simulink model "BPSK_EXP3"  (R2020a)
settings: Solver=VariableStepAuto  StartTime=0.0  StopTime=15  RelTol=1e-3
libraries: commrandsrc3 x1, dsparch4 x1
settings Model: Creator=User  LastModifiedBy=Raksha

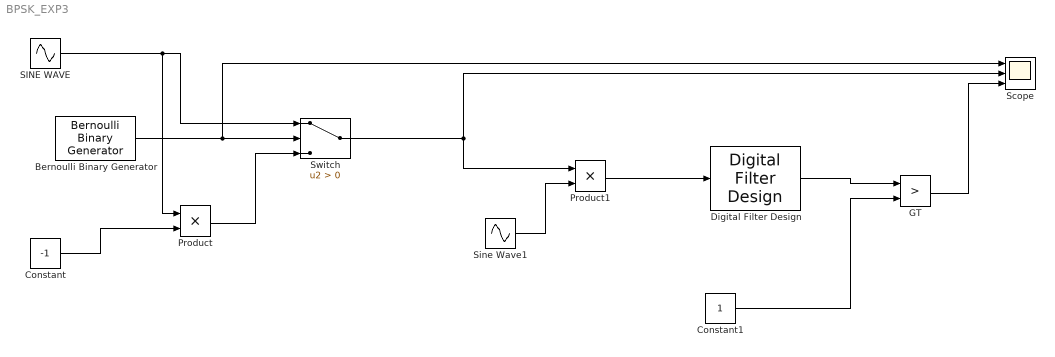
== system BPSK_EXP3 ==
  Bernoulli Binary Generator : commrandsrc3/Bernoulli Binary Generator  ProbabilityOfZero=0.5  SeedSource=Auto  Seed=0  SampleTime=1  SamplesPerFrame=1  OutputDataType=double  SimulateUsing=Interpreted execution
  Constant : Constant  Value=-1
  Constant1 : Constant
  Digital Filter Design : dsparch4/Digital Filter Design  mwdsp_browser_bugfix_var=off
  GT : RelationalOperator  Operator=>  OutDataTypeStr=boolean  RndMeth=Simplest
  Product : Product
  Product1 : Product
  "SINE WAVE " : Sin  Amplitude=2  Frequency=4*pi  SampleTime=0.01
  Scope : Scope  NumInputPorts=3
  Sine Wave1 : Sin  Amplitude=4  Frequency=10  SampleTime=0.01
  Switch : Switch  Criteria=u2 > Threshold
  wires:
  "SINE WAVE "/1 -> Product/1, Switch/1
  Bernoulli Binary Generator/1 -> Scope/1, Switch/2
  Constant/1 -> Product/2
  Product/1 -> Switch/3
  Switch/1 -> Product1/1, Scope/2
  Sine Wave1/1 -> Product1/2
  Product1/1 -> Digital Filter Design/1
  Constant1/1 -> GT/2
  Digital Filter Design/1 -> GT/1
  GT/1 -> Scope/3
